simulink model "PPI_loops_rcac"  (R2023a)
settings: Solver=VariableStepAuto  StartTime=0.0  StopTime=T  FixedStep=time_step/10  RelTol=1e-3
values from neighbouring files (symbols this model uses):
  A = [zeros(3,3),eye(3);zeros(3,3),zeros(3,3)]    [calculate_gains.m]
  alpha_inner = alphas(i,1)    [loops_runner.m]    (also in loops_runner_invert_beta.m)
  alpha_outer = alphas(i,2)    [loops_runner.m]    (also in loops_runner_invert_beta.m)
  B = [zeros(3,3);diag([1/m,1/m,1/m])]    [calculate_gains.m]
  C = eye(6)    [calculate_gains.m]
  C_q = C_r    [calculate_gains.m]
  C_r = C(1:3,:)    [calculate_gains.m]
  C_v = C(4:6,:)    [calculate_gains.m]
  C_w = C_v    [calculate_gains.m]
  g = [0; 0; 10]    [calculate_gains.m]
  Jx = 0.005    [calculate_gains.m]
  Jy = 0.005    [calculate_gains.m]
  Jz = 0.009    [calculate_gains.m]
  Ka_il = 0.0    (= 0)    [loops_runner.m]    (also in loops_runner_invert_beta.m)
  Ka_ol = 1.0    (= 1)    [loops_runner.m]    (also in loops_runner_invert_beta.m)
  Ki2_IL = diag(ki)    [calculate_gains.m]
  Ki2_OL = eye(3)*ki2    [calculate_gains.m]
  Kp1_IL = diag(kr)    [calculate_gains.m]
  Kp1_OL = eye(3)*kp1    [calculate_gains.m]
  Kp2_IL = diag(kv)    [calculate_gains.m]
  Kp2_OL = eye(3)*kp2    [calculate_gains.m]
  rcac_att_ppi = struct('Ru_xy', 1.0,                 'Nf_xy', -1.0,                 'P0_xy', 0.1,                 'Ru_z', 1.0,                 'Nf_z', -1.0,                 'P0_z', 0.1,                 'PID', 1,                 'P0_id',0.0005,                 'N_id', 1,                 'eta', 0.1,                 'tau1', 40,                 'tau2', 200)    [loops_runner.m]    (also in loops_runner_invert_beta.m = struct('Ru_xy', 1.0,                 'Nf_xy', -1.0,         )
  rcac_pos_ppi = struct('Ru_xy', 0.005,                 'Nf_xy', -0.005,                 'P0_xy', 0.01,                 'Ru_z', 0.005,                 'Nf_z', -0.005,                 'P0_z', 0.005,                 'PID', 1,                 'P0_id',0.0005,                 'N_id', 1,                 'eta', 0.1,                 'tau1', 40,                 'tau2', 200)    [loops_runner.m]    (also in loops_runner_invert_beta.m = struct('Ru_xy', 0.01,                 'Nf_xy', -0.01/2,     )
  rcac_rate_ppi = struct('Ru_xy', 1.0,                 'Nf_xy', -1.0,                 'P0_xy', 0.000001,                 'Ru_z', 1.0,                 'Nf_z', -1.0,                 'P0_z', 0.000001,                 'PID', 2,                 'P0_id',0.0005,                 'N_id', 1,                 'eta', 0.1,                 'tau1', 40,                 'tau2', 200)    [loops_runner.m]    (also in loops_runner_invert_beta.m)
  rcac_vel_ppi = struct('Ru_xy', 1.0,                 'Nf_xy', -1.0,                 'P0_xy', 0.01,                 'Ru_z', 1.0,                 'Nf_z', -1.0,                 'P0_z', 0.001,                 'PID', 2,                 'P0_id',0.0005,                 'N_id', 1,                 'eta', 0.1,                 'tau1', 40,                 'tau2', 200)    [loops_runner.m]    (also in loops_runner_invert_beta.m = struct('Ru_xy', 0.01,                 'Nf_xy', -1.0/2,      )
  simin = timeseries(Traj,time)    [loops_runner.m]    (also in loops_runner_invert_beta.m)
  tau_m = 1/16    (= 0.0625)    [loops_runner.m]    (also in loops_runner_invert_beta.m)
  time_step = 0.001    [calculate_gains.m]
undefined symbols (not defined in the file or in its folder): DiscIntNeverNeededParam
libraries: simulink x1
settings Model: Creator=ankit  LastModifiedBy=yinyo
settings DataIOCC: SaveOutput=off  SignalLogging=off  DSMLogging=off
settings ModelReferenceCC: EnableRefExpFcnMdlSchedulingChecks=on

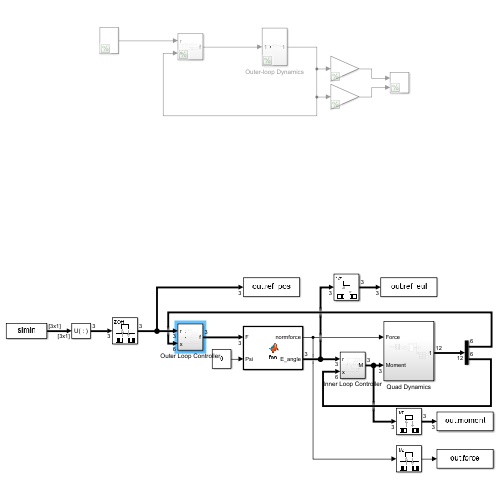
[thumbnail: Simulink's stored preview of the top-level diagram]
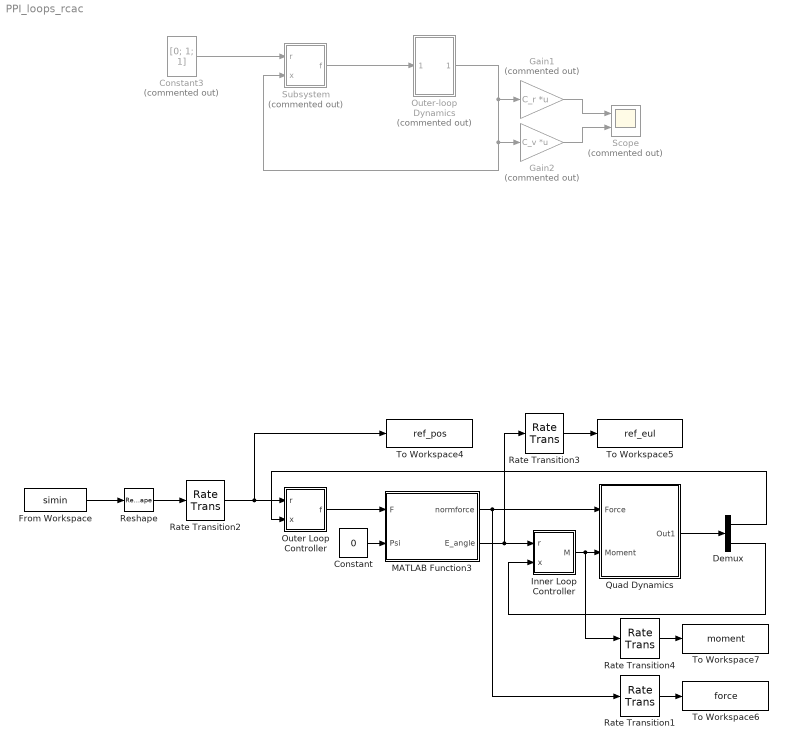
== system PPI_loops_rcac ==
  Constant : Constant  Value=0  SampleTime=time_step
  Constant3 : Constant  Commented=on  Value=[0; 1; 1]
  Demux : Demux  Outputs=[6 6]
  From Workspace : FromWorkspace  VariableName=simin
  Gain1 : Gain  Commented=on  Gain=C_r  Multiplication=Matrix(K*u)
  Gain2 : Gain  Commented=on  Gain=C_v  Multiplication=Matrix(K*u)
  Inner Loop Controller : Subsystem
  MATLAB Function3 : MATLAB Function  TreatAsAtomicUnit=on
  Outer Loop Controller : Subsystem
  Outer-loop Dynamics : Subsystem  Commented=on
  Quad Dynamics : Subsystem
  Rate Transition1 : RateTransition  OutPortSampleTime=0
  Rate Transition2 : RateTransition  InitialCondition=[squeeze(simin.Data(:,:,1))]'  OutPortSampleTime=time_step
  Rate Transition3 : RateTransition  InitialCondition=[0 0 0]  OutPortSampleTime=0
  Rate Transition4 : RateTransition  InitialCondition=[0 0 0]  OutPortSampleTime=0
  Reshape : Reshape
  Scope : Scope  Commented=on  NumInputPorts=2
  Subsystem : Subsystem  Commented=on
  To Workspace4 : ToWorkspace  VariableName=ref_pos  SampleTime=-1
  To Workspace5 : ToWorkspace  VariableName=ref_eul  SampleTime=-1
  To Workspace6 : ToWorkspace  VariableName=force  SampleTime=-1
  To Workspace7 : ToWorkspace  VariableName=moment  SampleTime=-1
  wires:
  Gain2/1 -> Scope/2
  Gain1/1 -> Scope/1
  Constant3/1 -> Subsystem/1(r)
  Outer-loop Dynamics/1(Out1) -> Subsystem/2(x), Gain2/1, Gain1/1
  Subsystem/1(f) -> Outer-loop Dynamics/1(In1)
  Inner Loop Controller/1(M) -> Rate Transition4/1, Quad Dynamics/2(Moment)
  MATLAB Function3/2(E_angle) -> Rate Transition3/1, Inner Loop Controller/1(r)
  MATLAB Function3/1(normforce) -> Quad Dynamics/1(Force), Rate Transition1/1
  Quad Dynamics/1(Out1) -> Demux/1
  Constant/1 -> MATLAB Function3/2(Psi)
  Outer Loop Controller/1(f) -> MATLAB Function3/1(F)
  Demux/1 -> Outer Loop Controller/2(x)
  Demux/2 -> Inner Loop Controller/2(x)
  From Workspace/1 -> Reshape/1
  Reshape/1 -> Rate Transition2/1
  Rate Transition2/1 -> To Workspace4/1, Outer Loop Controller/1(r)
  Rate Transition3/1 -> To Workspace5/1
  Rate Transition1/1 -> To Workspace6/1
  Rate Transition4/1 -> To Workspace7/1

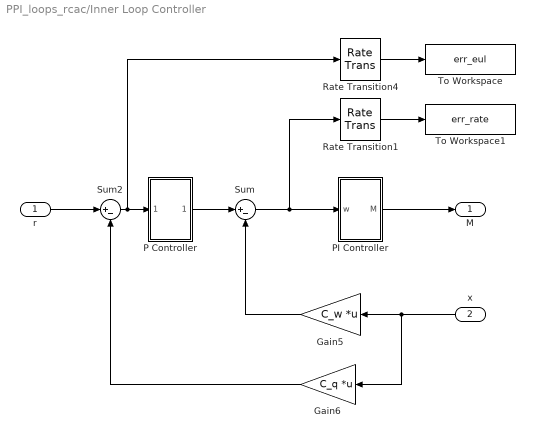
== system PPI_loops_rcac/Inner Loop Controller ==
  r : Inport
  x : Inport  Port=2
  Gain5 : Gain  Gain=C_w  Multiplication=Matrix(K*u)
  Gain6 : Gain  Gain=C_q  Multiplication=Matrix(K*u)
  P Controller : Subsystem
  PI Controller : Subsystem
  Rate Transition1 : RateTransition  InitialCondition=[0 0 0]  OutPortSampleTime=0
  Rate Transition4 : RateTransition  InitialCondition=[0 0 0]  OutPortSampleTime=0
  Sum : Sum  Inputs=|+-
  Sum2 : Sum  Inputs=|+-
  To Workspace : ToWorkspace  VariableName=err_eul  SampleTime=-1
  To Workspace1 : ToWorkspace  VariableName=err_rate  SampleTime=-1
  M : Outport
  wires:
  x/1 -> Gain6/1, Gain5/1
  Sum/1 -> Rate Transition1/1, PI Controller/1(w)
  P Controller/1(w_d) -> Sum/1
  Gain6/1 -> Sum2/2
  r/1 -> Sum2/1
  Gain5/1 -> Sum/2
  Sum2/1 -> Rate Transition4/1, P Controller/1(e_q)
  PI Controller/1(M) -> M/1
  Rate Transition4/1 -> To Workspace/1
  Rate Transition1/1 -> To Workspace1/1

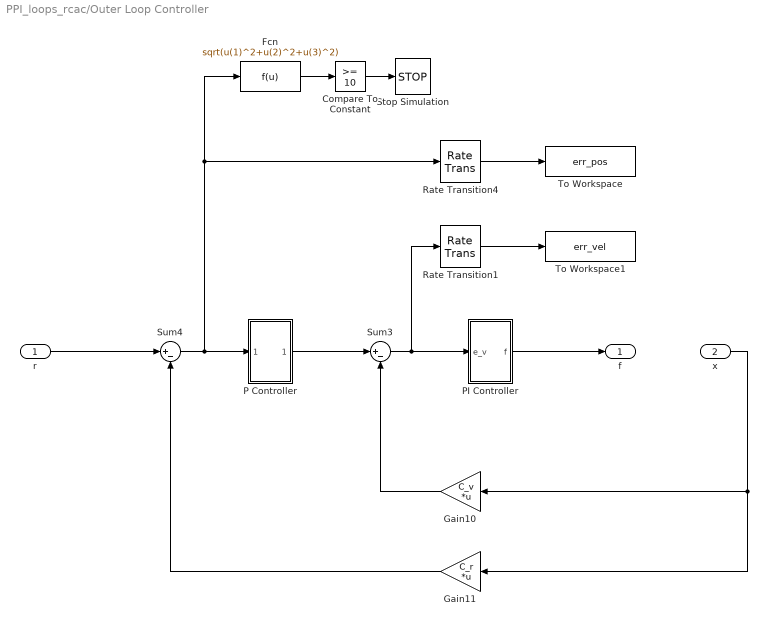
== system PPI_loops_rcac/Outer Loop Controller ==
  r : Inport
  x : Inport  Port=2
  Compare To Constant : simulink/Logic and Bit Operations/Compare To Constant  relop=>=  const=10  OutDataTypeStr=boolean
  Fcn : Fcn  Expr=sqrt(u(1)^2+u(2)^2+u(3)^2)
  Gain10 : Gain  Gain=C_v  Multiplication=Matrix(K*u)
  Gain11 : Gain  Gain=C_r  Multiplication=Matrix(K*u)
  P Controller : Subsystem
  PI Controller : Subsystem
  Rate Transition1 : RateTransition  InitialCondition=[0 0 0]  OutPortSampleTime=0
  Rate Transition4 : RateTransition  InitialCondition=[0 0 0]  OutPortSampleTime=0
  Stop Simulation : Stop
  Sum3 : Sum  Inputs=|+-
  Sum4 : Sum  Inputs=|+-
  To Workspace : ToWorkspace  VariableName=err_pos  SampleTime=-1
  To Workspace1 : ToWorkspace  VariableName=err_vel  SampleTime=-1
  f : Outport
  wires:
  Gain11/1 -> Sum4/2
  P Controller/1(v_d) -> Sum3/1
  x/1 -> Gain11/1, Gain10/1
  Gain10/1 -> Sum3/2
  r/1 -> Sum4/1
  PI Controller/1(f) -> f/1
  Sum3/1 -> Rate Transition1/1, PI Controller/1(e_v)
  Sum4/1 -> Fcn/1, Rate Transition4/1, P Controller/1(e_r)
  Fcn/1 -> Compare To Constant/1
  Compare To Constant/1 -> Stop Simulation/1
  Rate Transition4/1 -> To Workspace/1
  Rate Transition1/1 -> To Workspace1/1

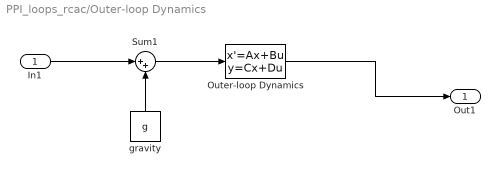
== system PPI_loops_rcac/Outer-loop Dynamics ==
  In1 : Inport
  Outer-loop Dynamics : StateSpace  A=A  B=B  C=C  D=zeros(6,3)  InitialCondition=0  ContinuousStateAttributes='position'
  Sum1 : Sum  Inputs=|++
  gravity : Constant  Value=g
  Out1 : Outport
  wires:
  gravity/1 -> Sum1/2
  In1/1 -> Sum1/1
  Sum1/1 -> Outer-loop Dynamics/1
  Outer-loop Dynamics/1 -> Out1/1

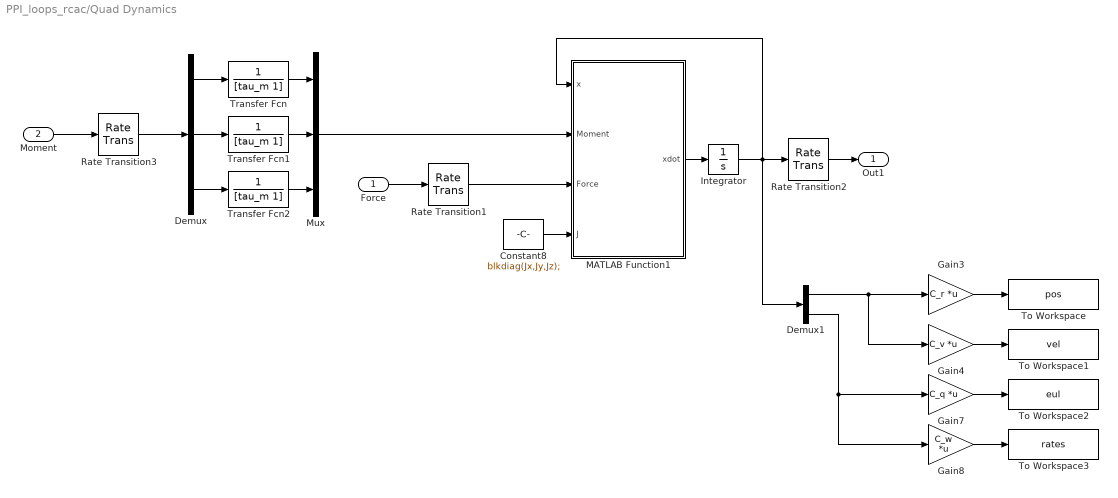
== system PPI_loops_rcac/Quad Dynamics ==
  Force : Inport
  Moment : Inport  Port=2
  Constant8 : Constant  Value=blkdiag(Jx,Jy,Jz);
  Demux : Demux  Outputs=3
  Demux1 : Demux  Outputs=[6 6]
  Gain3 : Gain  Gain=C_r  Multiplication=Matrix(K*u)
  Gain4 : Gain  Gain=C_v  Multiplication=Matrix(K*u)
  Gain7 : Gain  Gain=C_q  Multiplication=Matrix(K*u)
  Gain8 : Gain  Gain=C_w  Multiplication=Matrix(K*u)
  Integrator : Integrator
  MATLAB Function1 : MATLAB Function  TreatAsAtomicUnit=on
  Mux : Mux  Inputs=3
  Rate Transition1 : RateTransition  OutPortSampleTime=0
  Rate Transition2 : RateTransition  InitialCondition=zeros(1,12)  OutPortSampleTime=time_step
  Rate Transition3 : RateTransition  InitialCondition=[0 0 0]  OutPortSampleTime=0
  To Workspace : ToWorkspace  VariableName=pos  SampleTime=-1
  To Workspace1 : ToWorkspace  VariableName=vel  SampleTime=-1
  To Workspace2 : ToWorkspace  VariableName=eul  SampleTime=-1
  To Workspace3 : ToWorkspace  VariableName=rates  SampleTime=-1
  Transfer Fcn : TransferFcn  Denominator=[tau_m 1]
  Transfer Fcn1 : TransferFcn  Denominator=[tau_m 1]
  Transfer Fcn2 : TransferFcn  Denominator=[tau_m 1]
  Out1 : Outport
  wires:
  Constant8/1 -> MATLAB Function1/4(J)
  MATLAB Function1/1(xdot) -> Integrator/1
  Integrator/1 -> Demux1/1, Rate Transition2/1, MATLAB Function1/1(x)
  Force/1 -> Rate Transition1/1
  Moment/1 -> Rate Transition3/1
  Demux/1 -> Transfer Fcn/1
  Demux/2 -> Transfer Fcn1/1
  Demux/3 -> Transfer Fcn2/1
  Transfer Fcn1/1 -> Mux/2
  Transfer Fcn/1 -> Mux/1
  Transfer Fcn2/1 -> Mux/3
  Mux/1 -> MATLAB Function1/2(Moment)
  Rate Transition2/1 -> Out1/1
  Rate Transition1/1 -> MATLAB Function1/3(Force)
  Rate Transition3/1 -> Demux/1
  Demux1/1 -> Gain4/1, Gain3/1
  Gain7/1 -> To Workspace2/1
  Gain4/1 -> To Workspace1/1
  Gain8/1 -> To Workspace3/1
  Gain3/1 -> To Workspace/1
  Demux1/2 -> Gain7/1, Gain8/1

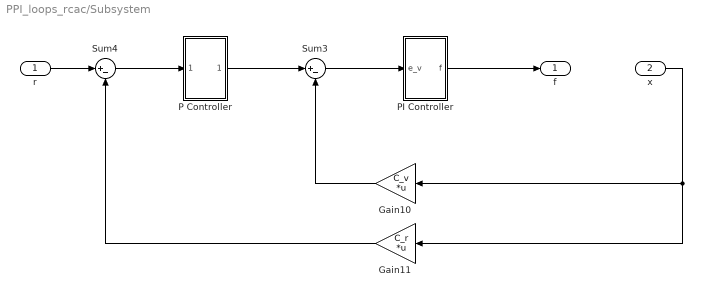
== system PPI_loops_rcac/Subsystem ==
  r : Inport
  x : Inport  Port=2
  Gain10 : Gain  Gain=C_v  Multiplication=Matrix(K*u)
  Gain11 : Gain  Gain=C_r  Multiplication=Matrix(K*u)
  P Controller : Subsystem
  PI Controller : Subsystem
  Sum3 : Sum  Inputs=|+-
  Sum4 : Sum  Inputs=|+-
  f : Outport
  wires:
  Gain11/1 -> Sum4/2
  P Controller/1(v_d) -> Sum3/1
  x/1 -> Gain11/1, Gain10/1
  Gain10/1 -> Sum3/2
  r/1 -> Sum4/1
  Sum4/1 -> P Controller/1(e_r)
  Sum3/1 -> PI Controller/1(e_v)
  PI Controller/1(f) -> f/1

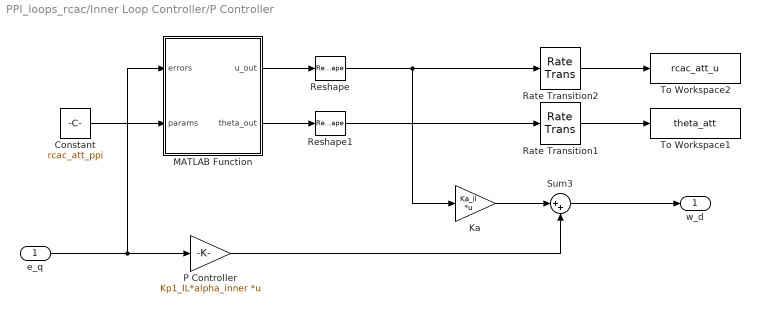
== system PPI_loops_rcac/Inner Loop Controller/P Controller ==
  e_q : Inport
  Constant : Constant  Value=rcac_att_ppi  OutDataTypeStr=Bus: RCACParamsBus
  Ka : Gain  Gain=Ka_il  Multiplication=Matrix(K*u)
  MATLAB Function : MATLAB Function  TreatAsAtomicUnit=on
  P Controller : Gain  Gain=Kp1_IL*alpha_inner  Multiplication=Matrix(K*u)
  Rate Transition1 : RateTransition  InitialCondition=zeros(1,3)  OutPortSampleTime=0
  Rate Transition2 : RateTransition  InitialCondition=[0 0 0]  OutPortSampleTime=0
  Reshape : Reshape
  Reshape1 : Reshape
  Sum3 : Sum  Inputs=|++
  To Workspace1 : ToWorkspace  VariableName=theta_att  SampleTime=-1
  To Workspace2 : ToWorkspace  VariableName=rcac_att_u  SampleTime=-1
  w_d : Outport
  wires:
  MATLAB Function/1(u_out) -> Reshape/1
  Rate Transition2/1 -> To Workspace2/1
  Reshape1/1 -> Rate Transition1/1
  Rate Transition1/1 -> To Workspace1/1
  Reshape/1 -> Ka/1, Rate Transition2/1
  MATLAB Function/2(theta_out) -> Reshape1/1
  e_q/1 -> MATLAB Function/1(errors), P Controller/1
  P Controller/1 -> Sum3/2
  Sum3/1 -> w_d/1
  Constant/1 -> MATLAB Function/2(params)
  Ka/1 -> Sum3/1

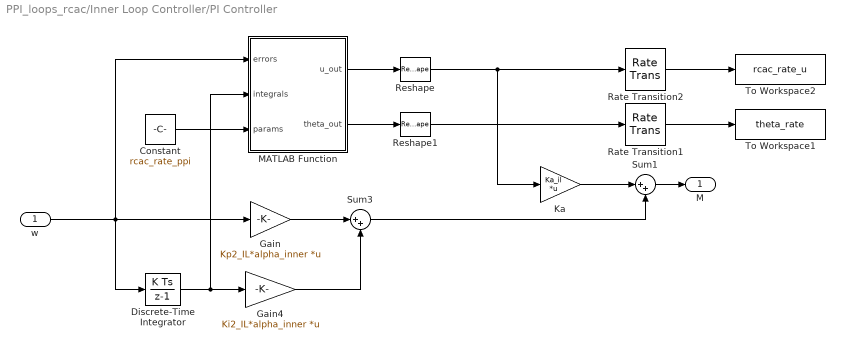
== system PPI_loops_rcac/Inner Loop Controller/PI Controller ==
  w : Inport
  Constant : Constant  Value=rcac_rate_ppi  OutDataTypeStr=Bus: RCACParamsBus
  Discrete-Time Integrator : DiscreteIntegrator  InitialCondition=[0 0 0]  SampleTime=time_step  ICPrevOutput=DiscIntNeverNeededParam  ICPrevScaledInput=DiscIntNeverNeededParam
  Gain : Gain  Gain=Kp2_IL*alpha_inner  Multiplication=Matrix(K*u)
  Gain4 : Gain  Gain=Ki2_IL*alpha_inner  Multiplication=Matrix(K*u)
  Ka : Gain  Gain=Ka_il  Multiplication=Matrix(K*u)
  MATLAB Function : MATLAB Function  TreatAsAtomicUnit=on
  Rate Transition1 : RateTransition  InitialCondition=zeros(1,6)  OutPortSampleTime=0
  Rate Transition2 : RateTransition  InitialCondition=[0 0 0]  OutPortSampleTime=0
  Reshape : Reshape
  Reshape1 : Reshape
  Sum1 : Sum  Inputs=|++
  Sum3 : Sum  Inputs=|++
  To Workspace1 : ToWorkspace  VariableName=theta_rate  SampleTime=-1
  To Workspace2 : ToWorkspace  VariableName=rcac_rate_u  SampleTime=-1
  M : Outport
  wires:
  Gain/1 -> Sum3/1
  Gain4/1 -> Sum3/2
  Rate Transition1/1 -> To Workspace1/1
  Reshape1/1 -> Rate Transition1/1
  MATLAB Function/2(theta_out) -> Reshape1/1
  Discrete-Time Integrator/1 -> MATLAB Function/2(integrals), Gain4/1
  w/1 -> MATLAB Function/1(errors), Discrete-Time Integrator/1, Gain/1
  Reshape/1 -> Ka/1, Rate Transition2/1
  Rate Transition2/1 -> To Workspace2/1
  MATLAB Function/1(u_out) -> Reshape/1
  Sum3/1 -> Sum1/2
  Sum1/1 -> M/1
  Constant/1 -> MATLAB Function/3(params)
  Ka/1 -> Sum1/1

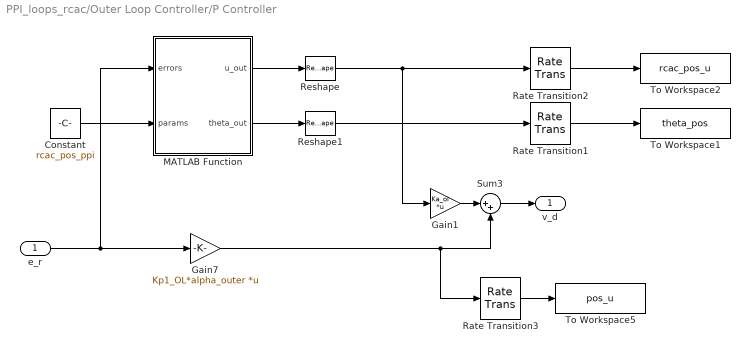
== system PPI_loops_rcac/Outer Loop Controller/P Controller ==
  e_r : Inport
  Constant : Constant  Value=rcac_pos_ppi  OutDataTypeStr=Bus: RCACParamsBus
  Gain1 : Gain  Gain=Ka_ol  Multiplication=Matrix(K*u)
  Gain7 : Gain  Gain=Kp1_OL*alpha_outer  Multiplication=Matrix(K*u)
  MATLAB Function : MATLAB Function  TreatAsAtomicUnit=on
  Rate Transition1 : RateTransition  InitialCondition=zeros(1,3)  OutPortSampleTime=0
  Rate Transition2 : RateTransition  InitialCondition=[0 0 0]  OutPortSampleTime=0
  Rate Transition3 : RateTransition  InitialCondition=[0 0 0]  OutPortSampleTime=0
  Reshape : Reshape
  Reshape1 : Reshape
  Sum3 : Sum  Inputs=|++
  To Workspace1 : ToWorkspace  VariableName=theta_pos  SampleTime=-1
  To Workspace2 : ToWorkspace  VariableName=rcac_pos_u  SampleTime=-1
  To Workspace5 : ToWorkspace  VariableName=pos_u  SampleTime=-1
  v_d : Outport
  wires:
  e_r/1 -> MATLAB Function/1(errors), Gain7/1
  Reshape/1 -> Gain1/1, Rate Transition2/1
  Reshape1/1 -> Rate Transition1/1
  MATLAB Function/2(theta_out) -> Reshape1/1
  Rate Transition2/1 -> To Workspace2/1
  MATLAB Function/1(u_out) -> Reshape/1
  Rate Transition1/1 -> To Workspace1/1
  Gain7/1 -> Rate Transition3/1, Sum3/2
  Sum3/1 -> v_d/1
  Constant/1 -> MATLAB Function/2(params)
  Gain1/1 -> Sum3/1
  Rate Transition3/1 -> To Workspace5/1

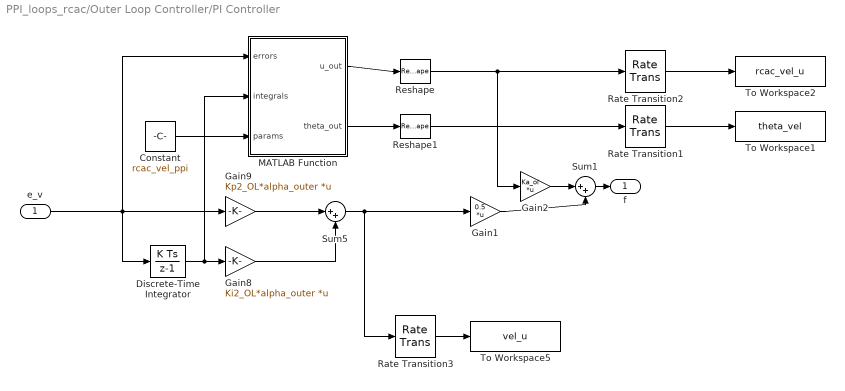
== system PPI_loops_rcac/Outer Loop Controller/PI Controller ==
  e_v : Inport
  Constant : Constant  Value=rcac_vel_ppi  OutDataTypeStr=Bus: RCACParamsBus
  Discrete-Time Integrator : DiscreteIntegrator  InitialCondition=[0 0 0]  SampleTime=time_step  ICPrevOutput=DiscIntNeverNeededParam  ICPrevScaledInput=DiscIntNeverNeededParam
  Gain1 : Gain  Gain=0.5  Multiplication=Matrix(K*u)
  Gain2 : Gain  Gain=Ka_ol  Multiplication=Matrix(K*u)
  Gain8 : Gain  Gain=Ki2_OL*alpha_outer  Multiplication=Matrix(K*u)
  Gain9 : Gain  Gain=Kp2_OL*alpha_outer  Multiplication=Matrix(K*u)
  MATLAB Function : MATLAB Function  TreatAsAtomicUnit=on
  Rate Transition1 : RateTransition  InitialCondition=zeros(1,6)  OutPortSampleTime=0
  Rate Transition2 : RateTransition  InitialCondition=[0 0 0]  OutPortSampleTime=0
  Rate Transition3 : RateTransition  InitialCondition=[0 0 0]  OutPortSampleTime=0
  Reshape : Reshape
  Reshape1 : Reshape
  Sum1 : Sum  Inputs=|++
  Sum5 : Sum  Inputs=|++
  To Workspace1 : ToWorkspace  VariableName=theta_vel  SampleTime=-1
  To Workspace2 : ToWorkspace  VariableName=rcac_vel_u  SampleTime=-1
  To Workspace5 : ToWorkspace  VariableName=vel_u  SampleTime=-1
  f : Outport
  wires:
  Gain9/1 -> Sum5/1
  Discrete-Time Integrator/1 -> MATLAB Function/2(integrals), Gain8/1
  e_v/1 -> Discrete-Time Integrator/1, MATLAB Function/1(errors), Gain9/1
  Gain8/1 -> Sum5/2
  Rate Transition1/1 -> To Workspace1/1
  Rate Transition2/1 -> To Workspace2/1
  Sum5/1 -> Rate Transition3/1, Gain1/1
  Rate Transition3/1 -> To Workspace5/1
  MATLAB Function/1(u_out) -> Reshape/1
  MATLAB Function/2(theta_out) -> Reshape1/1
  Reshape/1 -> Gain2/1, Rate Transition2/1
  Reshape1/1 -> Rate Transition1/1
  Sum1/1 -> f/1
  Gain1/1 -> Sum1/2
  Constant/1 -> MATLAB Function/3(params)
  Gain2/1 -> Sum1/1

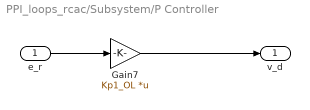
== system PPI_loops_rcac/Subsystem/P Controller ==
  e_r : Inport
  Gain7 : Gain  Gain=Kp1_OL  Multiplication=Matrix(K*u)
  v_d : Outport
  wires:
  Gain7/1 -> v_d/1
  e_r/1 -> Gain7/1

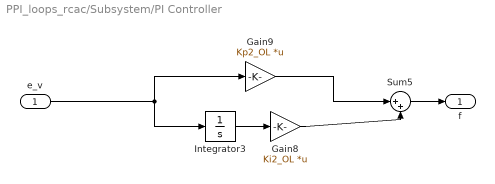
== system PPI_loops_rcac/Subsystem/PI Controller ==
  e_v : Inport
  Gain8 : Gain  Gain=Ki2_OL  Multiplication=Matrix(K*u)
  Gain9 : Gain  Gain=Kp2_OL  Multiplication=Matrix(K*u)
  Integrator3 : Integrator
  Sum5 : Sum  Inputs=|++
  f : Outport
  wires:
  Gain9/1 -> Sum5/1
  Integrator3/1 -> Gain8/1
  Sum5/1 -> f/1
  e_v/1 -> Gain9/1, Integrator3/1
  Gain8/1 -> Sum5/2

== matlab function PPI_loops_rcac/Outer Loop Controller/PI Controller/MATLAB Function ==
  data: u_out output; errors input; integrals input; theta_out output; params input
function [u_out, theta_out] = rcac_step(errors, integrals, params)
%% Persistent variables
persistent iter
persistent u_k
persistent theta P_blk ubar Phibar_blk 

if isempty(iter)
    iter = 1;
    u_k = zeros(3,1);
    ubar = zeros(2,3);
    P_blk = zeros(2,2,3);
    Phibar_blk = zeros(3,2,3);
    theta = zeros(2,3);
end

%% Constants
Rz_xy = 1.0;
Ru_xy = params.Ru_xy;
Nf_xy = params.Nf_xy;
P0_xy = params.P0_xy;

Rz_z = 1.0;
Ru_z = params.Ru_z;
Nf_z = params.Nf_z;
P0_z = params.P0_z;

errorNormMode = 0;

%% Run RCAC loop
for ii = 1:3
    % Set RCAC params according to axes
    if ii<3
       P0_val = P0_xy;
       Rz = Rz_xy;
       Ru = Ru_xy;
       Nf = Nf_xy;
    else
       P0_val = P0_z;
       Rz = Rz_z;
       Ru = Ru_z;
       Nf = Nf_z;
    end
    
    % build phi block
    phi_in = [errors(ii) integrals(ii)];

    % current state
    z_in = errors(ii);

    % Run rcac step function
    [u_k(ii), theta(:,ii),  P_blk(:,:,ii), ubar(:,ii), Phibar_blk(:,:,ii)] = RCAC_Step(iter, u_k(ii), z_in, phi_in, P0_val, Rz, Ru, Nf, errorNormMode, squeeze(P_blk(:,:,ii)), theta(:,ii), ubar(:,ii), squeeze(Phibar_blk(:,:,ii)));

end

%% Increment
iter = iter + 1;

%% Output
u_out = u_k;
theta_out = [theta(:,1); theta(:,2); theta(:,3)];

end

== matlab function PPI_loops_rcac/Quad Dynamics/MATLAB Function1 ==
  data: x input; xdot output; Moment input; Force input; J input
function xdot  = rotation_dynam(x, Moment, Force, J)%xdot 6x1, u moment

xdot=zeros(12,1);
v = x(4:6,1);
omega_QE = x(10:12,1);

m=0.8;
moment= Moment;
force=Force;
g=[0;0;10];
phi=x(7);
theta=x(8);
psi=x(9);

[O3psi, O2theta, O1phi] = orientation_matrices(phi, theta, psi);
xdot(1:3,1) = v;
xdot(4:6,1) = g + force/m*transpose(O3psi) * transpose(O2theta) * transpose(O1phi)*[0;0;1];

xdot(7:9,1) = S_Phi_Theta(phi,theta)*omega_QE;
%phi/theta/psi dot

xdot(10:12,1) = J\(-cross(omega_QE,J*omega_QE)+moment);
%P/Q/R dot

function S = S_Phi_Theta(Phi,Theta)
S = [1 sin(Phi)*tan(Theta) cos(Phi)*tan(Theta);
    0 cos(Phi) -sin(Phi);
    0 sin(Phi)*sec(Theta) cos(Phi)*sec(Theta)];
end

function [O3psi, O2theta, O1phi] = orientation_matrices(phi, theta, psi);
O3psi = [cos(psi) sin(psi) 0;
    -sin(psi) cos(psi) 0;
    0 0 1];
O2theta = [cos(theta) 0 -sin(theta);
    0 1 0
    sin(theta) 0 cos(theta)];
O1phi = [1 0 0
    0 cos(phi) sin(phi);
    0 -sin(phi) cos(phi) ;];
end





end

== matlab function PPI_loops_rcac/Inner Loop Controller/PI Controller/MATLAB Function ==
  data: u_out output; errors input; integrals input; theta_out output; params input
function [u_out, theta_out] = rcac_step(errors, integrals, params)
%% Persistent variables
persistent iter
persistent u_k
persistent theta P_blk ubar Phibar_blk 

if isempty(iter)
    iter = 1;
    u_k = zeros(3,1);
    ubar = zeros(2,3);
    P_blk = zeros(2,2,3);
    Phibar_blk = zeros(3,2,3);
    theta = zeros(2,3);
end

%% Constants
Rz_xy = 1.0;
Ru_xy = params.Ru_xy;
Nf_xy = params.Nf_xy;
P0_xy = params.P0_xy;

Rz_z = 1.0;
Ru_z = params.Ru_z;
Nf_z = params.Nf_z;
P0_z = params.P0_z;

errorNormMode = 0;

%% Run RCAC loop
for ii = 1:3
    % Set RCAC params according to axes
    if ii<3
       P0_val = P0_xy;
       Rz = Rz_xy;
       Ru = Ru_xy;
       Nf = Nf_xy;
    else
       P0_val = P0_z;
       Rz = Rz_z;
       Ru = Ru_z;
       Nf = Nf_z;
    end
    
    % build phi block
    phi_in = [errors(ii) integrals(ii)];

    % current state
    z_in = errors(ii);

    % Run rcac step function
    [u_k(ii), theta(:,ii),  P_blk(:,:,ii), ubar(:,ii), Phibar_blk(:,:,ii)] = RCAC_Step(iter, u_k(ii), z_in, phi_in, P0_val, Rz, Ru, Nf, errorNormMode, squeeze(P_blk(:,:,ii)), theta(:,ii), ubar(:,ii), squeeze(Phibar_blk(:,:,ii)));
end

%% Increment
iter = iter + 1;

%% Output
u_out = u_k;
theta_out = [theta(:,1); theta(:,2); theta(:,3)];

end

== matlab function PPI_loops_rcac/MATLAB Function3 ==
  data: normforce output; F input; Psi input; E_angle output
function [normforce, E_angle] = fcn(F, Psi)

E_angle=zeros(3,1);
normforce=0;
para1=0;
para2=0;
fx=F(1);
fy=F(2);
fz=F(3);

magni=-sqrt(fx^2+fy^2+fz^2);
if magni==0
    psi=Psi;
    theta=0;
    phi=0;
    E_angle=[phi;theta;psi];
    normforce=0;

else
psi=Psi;
normforce=magni;

f1=fx/magni;
f2=fy/magni;
f3=fz/magni;

%O3*O2*O1
% phi=asin(f2);
% theta=acos(f3/cos(phi));

%Tranpose O3*O2*O1
% theta=asin(f1);
% phi=acos(f3/cos(theta));

%O1*O2*O3
% theta=-asin(f1);
% phi=asin(f2/cos(theta));

%tranpose O1*O2*O3

phi=-asin(f2);
if abs(phi) >= 8*pi/9
    if phi >= 0.0
        phi = 8*pi/9;
    else 
        phi = -8*pi/9;
    end
end

theta=asin(f1/cos(phi));


para1=f2;
para2=f1/cos(phi);
E_angle=[phi; theta; psi];

end

== matlab function PPI_loops_rcac/Outer Loop Controller/P Controller/MATLAB Function ==
  data: u_out output; errors input; theta_out output; params input
function [u_out, theta_out] = rcac_step(errors,params)
%% Persistent variables
persistent iter
persistent u_k
persistent theta P_blk ubar Phibar_blk 

l_theta = 1;

if isempty(iter)
    iter = 1;
    u_k = zeros(3,1);
    ubar = zeros(2,3);
    P_blk = zeros(l_theta,l_theta,3);
    Phibar_blk = zeros(3,l_theta,3);
    theta = zeros(l_theta,3);
end

%% Constants
Rz_xy = 1.0;
Ru_xy = params.Ru_xy;
Nf_xy = params.Nf_xy;
P0_xy = params.P0_xy;

Rz_z = 1.0;
Ru_z = params.Ru_z;
Nf_z = params.Nf_z;
P0_z = params.P0_z;

errorNormMode = 0;

%% Run RCAC loop
for ii = 1:3
    % Set RCAC params according to axes
    if ii<3
       P0_val = P0_xy;
       Rz = Rz_xy;
       Ru = Ru_xy;
       Nf = Nf_xy;
    else
       P0_val = P0_z;
       Rz = Rz_z;
       Ru = Ru_z;
       Nf = Nf_z;
    end
    
    % build phi block
    phi_in = [errors(ii)];

    % current state
    z_in = errors(ii);

    % Run rcac step function
    [u_k(ii), theta(:,ii),  P_blk(:,:,ii), ubar(:,ii), Phibar_blk(:,:,ii)] = RCAC_Step(iter, u_k(ii), z_in, phi_in, P0_val, Rz, Ru, Nf, errorNormMode, squeeze(P_blk(:,:,ii)), theta(:,ii), ubar(:,ii), squeeze(Phibar_blk(:,:,ii)));

end

%% Increment
iter = iter + 1;

%% Output
u_out = u_k;
theta_out = [theta(:,1); theta(:,2); theta(:,3)];

end

== matlab function PPI_loops_rcac/Inner Loop Controller/P Controller/MATLAB Function ==
  data: u_out output; errors input; theta_out output; params input
function [u_out, theta_out] = rcac_step(errors, params)
%% Persistent variables
persistent iter
persistent u_k
persistent theta P_blk ubar Phibar_blk 

l_theta = 1;

if isempty(iter)
    iter = 1;
    u_k = zeros(3,1);
    ubar = zeros(2,3);
    P_blk = zeros(l_theta,l_theta,3);
    Phibar_blk = zeros(3,l_theta,3);
    theta = zeros(l_theta,3);
end

%% Constants
Rz_xy = 1.0;
Ru_xy = params.Ru_xy;
Nf_xy = params.Nf_xy;
P0_xy = params.P0_xy;

Rz_z = 1.0;
Ru_z = params.Ru_z;
Nf_z = params.Nf_z;
P0_z = params.P0_z;

errorNormMode = 0;

%% Run RCAC loop
for ii = 1:3
    % Set RCAC params according to axes
    if ii<3
       P0_val = P0_xy;
       Rz = Rz_xy;
       Ru = Ru_xy;
       Nf = Nf_xy;
    else
       P0_val = P0_z;
       Rz = Rz_z;
       Ru = Ru_z;
       Nf = Nf_z;
    end
    
    % build phi block
    phi_in = [errors(ii)];

    % current state
    z_in = errors(ii);

    % Run rcac step function
    [u_k(ii), theta(:,ii),  P_blk(:,:,ii), ubar(:,ii), Phibar_blk(:,:,ii)] = RCAC_Step(iter, u_k(ii), z_in, phi_in, P0_val, Rz, Ru, Nf, errorNormMode, squeeze(P_blk(:,:,ii)), theta(:,ii), ubar(:,ii), squeeze(Phibar_blk(:,:,ii)));

end

%% Increment
iter = iter + 1;

%% Output
u_out = u_k;
theta_out = [theta(:,1); theta(:,2); theta(:,3)];

end
